simulink model "simulink_caso1"  (R2023a)
settings: Solver=VariableStepAuto  StartTime=0.0  StopTime=10.0  RelTol=1e-3
undefined symbols (not defined in the file): A, Aest, B, Best, C, Cest, D, Dest0, K0d, Kd, X0
libraries: simulink x1
settings Model: Creator=Agustin  LastModifiedBy=Agustin

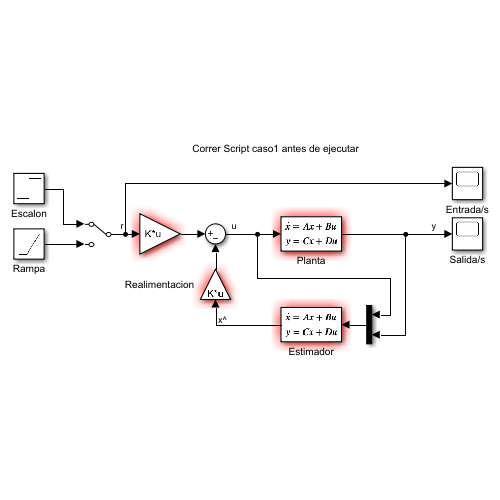
[thumbnail: Simulink's stored preview of the top-level diagram]
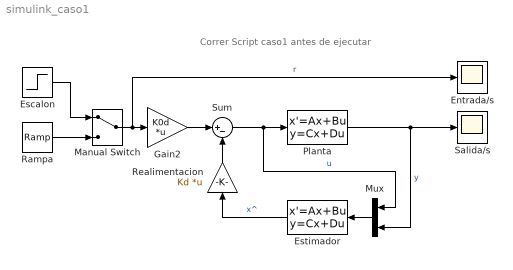
== system simulink_caso1 ==
  note: Correr Script caso1 antes de ejecutar
  Entrada/s : Scope
  Escalon : Step  SampleTime=0
  Estimador : StateSpace  A=Aest  B=Best  C=Cest  D=Dest0  InitialCondition=0
  Gain2 : Gain  Gain=K0d  Multiplication=Matrix(K*u)
  Manual Switch : ManualSwitch
  Mux : Mux  Inputs=2
  Planta : StateSpace  A=A  B=B  C=C  D=D  InitialCondition=X0
  Rampa : simulink/Sources/Ramp  slope=1  start=0  InitialOutput=0
  Realimentacion : Gain  Gain=Kd  Multiplication=Matrix(K*u)
  Salida/s : Scope
  Sum : Sum  Inputs=|+-
  wires:
  Planta/1 -> Mux/2, Salida/s/1  "y"
  Estimador/1 -> Realimentacion/1  "x^"
  Escalon/1 -> Manual Switch/1
  Realimentacion/1 -> Sum/2
  Sum/1 -> Mux/1, Planta/1  "u"
  Gain2/1 -> Sum/1
  Rampa/1 -> Manual Switch/2
  Manual Switch/1 -> Entrada/s/1, Gain2/1  "r"
  Mux/1 -> Estimador/1
